simulink model "Ereignisgenerator"  (R2014a)
settings: Solver=ode45  StartTime=0.0  StopTime=50  RelTol=1e-3
values from neighbouring files (symbols this model uses):
  EncoderDegree = 180    [DelayDensity_GeneticAlgorithm.m]
  Ereignisgenerator_Sampletime = 0.01    [DelayDensity_GeneticAlgorithm.m]
undefined symbols (not defined in the file or in its folder): des, gcbh
libraries: simulink x2
settings Model: Creator=shenc  LastModifiedBy=shenc

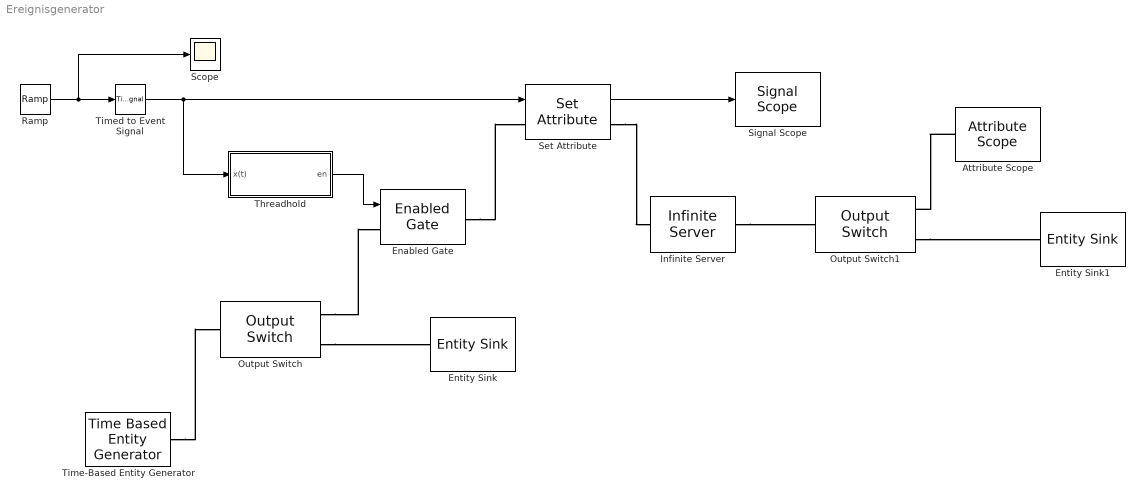
== system Ereignisgenerator ==
  Attribute Scope : AttributeScope  LoadFcn=des.scope.CallbackSupport('seLoadFcn',gcbh)  StartFcn=des.scope.CallbackSupport('seStartFcn',gcbh)  StopFcn=des.scope.CallbackSupport('seStopFcn',gcbh)  AttributeNameY=Value
      settings: CopyFcn=des.scope.CallbackSupport('seCopyFcn',gcbh)  DeleteFcn=des.scope.CallbackSupport('seDeleteFcn',gcbh)  PreSaveFcn=des.scope.CallbackSupport('sePreSaveFcn',gcbh)  NameChangeFcn=des.scope.CallbackSupport('seNameChangeFcn',gcbh)  OpenFcn=des.scope.CallbackSupport('seOpenFcn',gcbh)
  Enabled Gate : EnabledGate
  Entity Sink : EntitySink
  Entity Sink1 : EntitySink
  Infinite Server : InfiniteServer  ServiceTime=0.1
  Output Switch : OutputSwitch  NumberOutputPorts=2
  Output Switch1 : OutputSwitch  NumberOutputPorts=2
  Ramp : simulink/Sources/Ramp  slope=10  start=0  X0=0
  Scope : Scope
  Set Attribute : SetAttribute  AttributeName=Value  AttributeFrom=Signal port  StatNumberDeparted=on  EvaluatedAttributeValue={ []}
  Signal Scope : SignalScope  LoadFcn=des.scope.CallbackSupport('seLoadFcn',gcbh)  StartFcn=des.scope.CallbackSupport('seStartFcn',gcbh)  StopFcn=des.scope.CallbackSupport('seStopFcn',gcbh)
      settings: CopyFcn=des.scope.CallbackSupport('seCopyFcn',gcbh)  DeleteFcn=des.scope.CallbackSupport('seDeleteFcn',gcbh)  PreSaveFcn=des.scope.CallbackSupport('sePreSaveFcn',gcbh)  NameChangeFcn=des.scope.CallbackSupport('seNameChangeFcn',gcbh)  OpenFcn=des.scope.CallbackSupport('seOpenFcn',gcbh)
  Threadhold : Subsystem
  Time-Based Entity Generator : TimeBasedEntityGenerator  Period=Ereignisgenerator_Sampletime
  Timed to Event Signal : TimedToEventSignal
  wires:
  Ramp/1 -> Timed to Event Signal/1, Scope/1
  Threadhold/1(en) -> Enabled Gate/1
  Set Attribute/1 -> Signal Scope/1
  Timed to Event Signal/1 -> Set Attribute/1, Threadhold/1(x(t))
  connections:
  Time-Based Entity Generator/RConn1 -- Output Switch/LConn1
  Output Switch/RConn2 -- Entity Sink/LConn1
  Output Switch/RConn1 -- Enabled Gate/LConn1
  Enabled Gate/RConn1 -- Set Attribute/LConn1
  Set Attribute/RConn1 -- Infinite Server/LConn1
  Infinite Server/RConn1 -- Output Switch1/LConn1
  Output Switch1/RConn2 -- Entity Sink1/LConn1
  Attribute Scope/LConn1 -- Output Switch1/RConn1

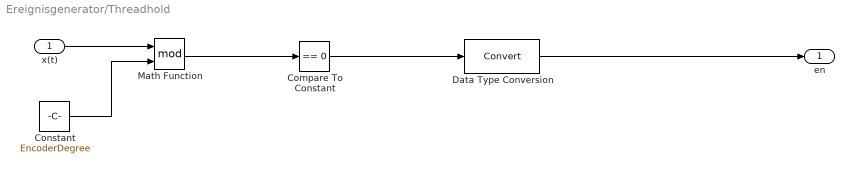
== system Ereignisgenerator/Threadhold ==
  x(t) : Inport
  Compare To Constant : simulink/Logic and Bit Operations/Compare To Constant  relop===  const=0  OutDataTypeStr=boolean
  Constant : Constant  Value=EncoderDegree
  Data Type Conversion : DataTypeConversion
  Math Function : Math  Operator=mod  SaturateOnIntegerOverflow=on
  en : Outport
  wires:
  x(t)/1 -> Math Function/1
  Constant/1 -> Math Function/2
  Math Function/1 -> Compare To Constant/1
  Compare To Constant/1 -> Data Type Conversion/1
  Data Type Conversion/1 -> en/1
